simulink model "mass_spring_damper"  (R2023b)
settings: Solver=VariableStepAuto  StartTime=0.0  StopTime=10.0  RelTol=1e-3
values from neighbouring files (symbols this model uses):
  A = 1    [Lab1_Es1.m]
  c = 1    [Lab1_Es1.m]
  f0 = 2*pi    (= 6.28318530718)    [Lab1_Es1.m]
  k = 1    [Lab1_Es1.m]
  K1 = 1/2 - 1i/2/sqrt(3)    [Lab1_Es1.m]
  K2 = 1/2 + 1i/2/sqrt(3)    [Lab1_Es1.m]
  m = 1    [Lab1_Es1.m]
  v0 = 0    [Lab1_Es1.m]
  x0 = 1    [Lab1_Es1.m]
libraries: simulink x1
settings Model: Creator=alberto  LastModifiedBy=alberto

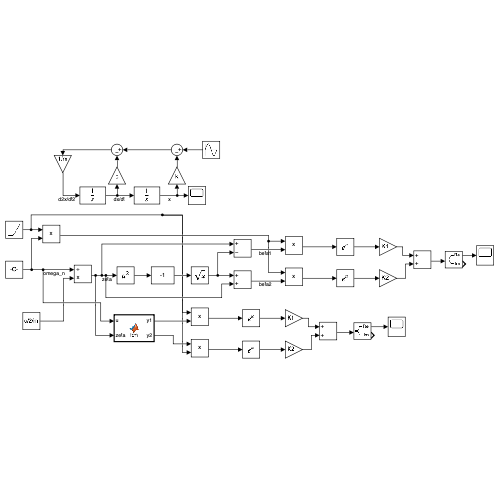
[thumbnail: Simulink's stored preview of the top-level diagram]
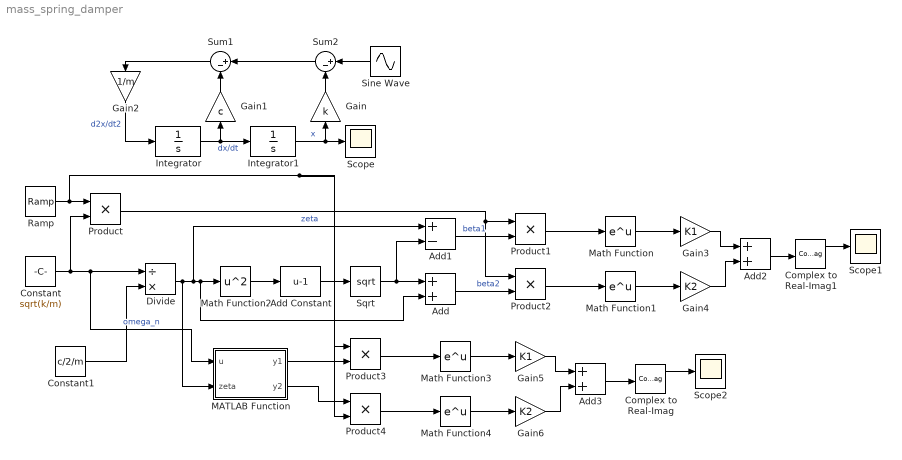
== system mass_spring_damper ==
  Add : Sum
  Add Constant : Bias  Bias=-1  SaturateOnIntegerOverflow=off
  Add1 : Sum  Inputs=+-
  Add2 : Sum
  Add3 : Sum
  Complex to Real-Imag : ComplexToRealImag
  Complex to Real-Imag1 : ComplexToRealImag
  Constant : Constant  Value=sqrt(k/m)
  Constant1 : Constant  Value=c/2/m
  Divide : Product  Inputs=/*
  Gain : Gain  Gain=k
  Gain1 : Gain  Gain=c
  Gain2 : Gain  Gain=1/m
  Gain3 : Gain  Gain=K1
  Gain4 : Gain  Gain=K2
  Gain5 : Gain  Gain=K1
  Gain6 : Gain  Gain=K2
  Integrator : Integrator  InitialCondition=v0
  Integrator1 : Integrator  InitialCondition=x0
  MATLAB Function : MATLAB Function  TreatAsAtomicUnit=on
  Math Function{,1,3..4} (4 alike) : Math
  Math Function2 : Math  Operator=square
  Product{,1..4} (5 alike) : Product
  Ramp : simulink/Sources/Ramp  slope=-1  start=0  InitialOutput=0
  Scope : Scope
  Scope1 : Scope
  Scope2 : Scope
  Sine Wave : Sin  Amplitude=A  Frequency=f0  SampleTime=0
  Sqrt : Sqrt  OutputSignalType=complex
  Sum1 : Sum  Inputs=|+-
  Sum2 : Sum  Inputs=|+-
  wires:
  Gain2/1 -> Integrator/1  "d2x/dt2"
  Integrator/1 -> Integrator1/1, Gain1/1  "dx/dt"
  Integrator1/1 -> Scope/1, Gain/1  "x"
  Gain1/1 -> Sum1/2
  Gain/1 -> Sum2/2
  Sine Wave/1 -> Sum2/1
  Sum2/1 -> Sum1/1
  Sum1/1 -> Gain2/1
  Constant/1 -> Product/2, Divide/1, MATLAB Function/1(u)  "omega_n"
  Divide/1 -> Add1/1, Add/2, Math Function2/1, MATLAB Function/2(zeta)  "zeta"
  Math Function2/1 -> Add Constant/1
  Add Constant/1 -> Sqrt/1
  Constant1/1 -> Divide/2
  Sqrt/1 -> Add1/2, Add/1
  Ramp/1 -> Product4/2, Product3/1, Product/1
  Add1/1 -> Product1/2  "beta1"
  Add/1 -> Product2/2  "beta2"
  Product/1 -> Product2/1, Product1/1
  Product1/1 -> Math Function/1
  Product2/1 -> Math Function1/1
  Math Function/1 -> Gain3/1
  Math Function1/1 -> Gain4/1
  Gain3/1 -> Add2/1
  Gain4/1 -> Add2/2
  Add2/1 -> Complex to Real-Imag1/1
  MATLAB Function/1(y1) -> Product3/2
  MATLAB Function/2(y2) -> Product4/1
  Product4/1 -> Math Function4/1
  Math Function4/1 -> Gain6/1
  Math Function3/1 -> Gain5/1
  Add3/1 -> Complex to Real-Imag/1
  Product3/1 -> Math Function3/1
  Gain6/1 -> Add3/2
  Gain5/1 -> Add3/1
  Complex to Real-Imag1/1 -> Scope1/1
  Complex to Real-Imag/1 -> Scope2/1

== matlab function mass_spring_damper/MATLAB Function ==
  data: u input; y1 output; zeta input; y2 output
function [y1, y2] = fcn(u, zeta)

app_var =sqrt(complex(zeta^2-1));
y1 = u * (zeta + app_var);
y2 = u * (zeta - app_var);
